simulink model "TailsitterSimModel_ArduPilot_SITL"  (R2018b)
settings: Solver=ode23  StartTime=0  StopTime=1200  FixedStep=0.01  RelTol=1e-4  EnableMultiTasking=on
undefined symbols (not defined in the file): envir
libraries: unit_conversions_lib x3, tailsitter_lib x2, ardupilot_sitl_lib x2, atmosphere_lib x1, flightgear_visualization_lib x1, actuators_lib x1, sensors_lib x1
settings Model: EnablePacing=on  Creator=Yannic  LastModifiedBy=yannic
settings SolverCC: ZeroCrossControl=DisableAll  AlgebraicLoopSolver=LineSearch
settings DataIOCC: LimitDataPoints=on  SaveFormat=StructureWithTime
settings OptimizationCC: BlockReduction=off  DefaultParameterBehavior=Inlined  DefaultUnderspecifiedDataType=single  OptimizeBlockIOStorage=off  BufferReuse=off  GlobalBufferReuse=off  ExpressionFolding=off  LocalBlockOutputs=off  LifeSpan=inf  OptimizeDataStoreBuffers=off  BusAssignmentInplaceUpdate=off
settings DebuggingCC: AlgebraicLoopMsg=none  UnconnectedInputMsg=none  UnconnectedOutputMsg=none  UnconnectedLineMsg=none  AllowSymbolicDim=off  SFUnexpectedBacktrackingDiag=warning  SFNoUnconditionalDefaultTransitionDiag=warning  SFExecutionAtInitializationDiag=none
settings ModelReferenceCC: PropagateSignalLabelsOutOfModel=off
settings SFSimCC: SimUseLocalCustomCode=off
settings RTWCC: RTWUseLocalCustomCode=off
settings CodeAppCC: StateflowObjectComments=on
settings GRTTargetCC: TargetLangStandard=C89/C90 (ANSI)
settings ConfigComp: CovMetricSettings=dw  CovHtmlReporting=on  CovSaveCumulativeToWorkspaceVar=on  CovSaveSingleToWorkspaceVar=on  CovExternalEMLEnable=off

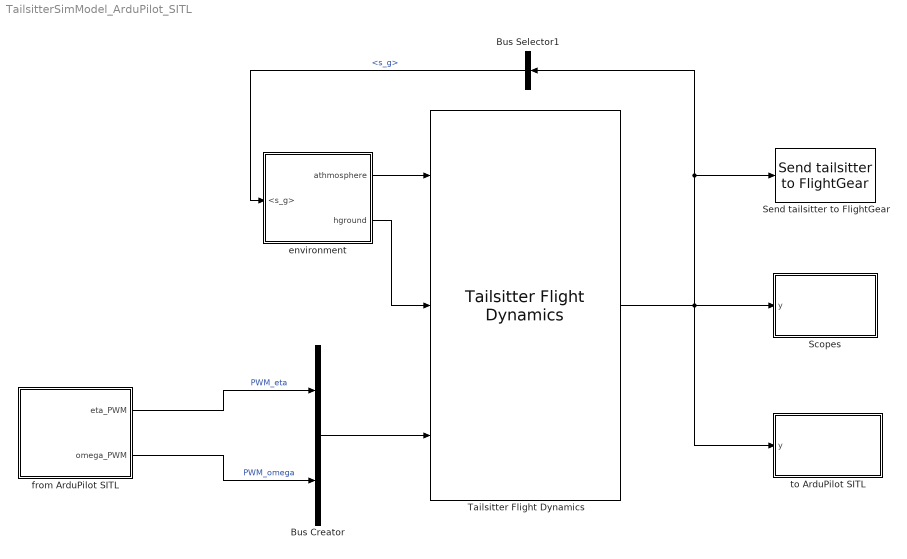
== system TailsitterSimModel_ArduPilot_SITL ==
  Bus Creator : BusCreator  Inputs=2
  Bus Selector1 : BusSelector  OutputSignals=rigid_body.s_g
  Scopes : Subsystem
  Send tailsitter to FlightGear : tailsitter_lib/Send tailsitter to FlightGear  posRef=tailsitter.posRef  IP='127.0.0.1'  Port=5502
      settings: SourceProductName=LADAC
  Tailsitter Flight Dynamics : tailsitter_lib/Tailsitter Flight Dynamics  tailsitter=tailsitter
      settings: SourceProductName=LADAC
  environment : Subsystem
  from ArduPilot SITL : Subsystem
  to ArduPilot SITL : Subsystem
  wires:
  from ArduPilot SITL/2(omega_PWM) -> Bus Creator/2  "PWM_omega"
  from ArduPilot SITL/1(eta_PWM) -> Bus Creator/1  "PWM_eta"
  Bus Creator/1 -> Tailsitter Flight Dynamics/3
  environment/1(athmosphere) -> Tailsitter Flight Dynamics/1
  environment/2(hground) -> Tailsitter Flight Dynamics/2
  Tailsitter Flight Dynamics/1 -> Send tailsitter to FlightGear/1, Bus Selector1/1, Scopes/1(y), to ArduPilot SITL/1(y)
  Bus Selector1/1 -> environment/1(<s_g>)  "<s_g>"

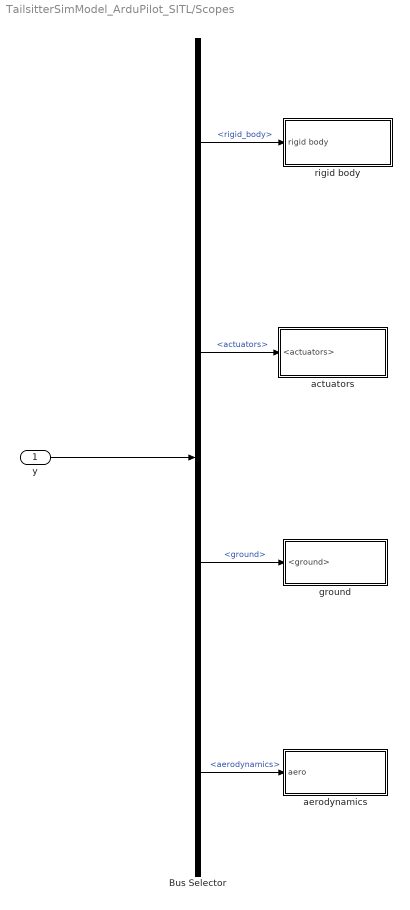
== system TailsitterSimModel_ArduPilot_SITL/Scopes ==
  y : Inport
  Bus Selector : BusSelector  OutputSignals=rigid_body,actuators,ground,aerodynamics
  actuators : Subsystem
  aerodynamics : Subsystem
  ground : Subsystem
  rigid body : Subsystem
  wires:
  Bus Selector/1 -> rigid body/1(rigid body)  "<rigid_body>"
  y/1 -> Bus Selector/1
  Bus Selector/4 -> aerodynamics/1(aero)  "<aerodynamics>"
  Bus Selector/3 -> ground/1(<ground>)  "<ground>"
  Bus Selector/2 -> actuators/1(<actuators>)  "<actuators>"

== system TailsitterSimModel_ArduPilot_SITL/environment ==
  <s_g> : Inport
  Atmosphere1 : Subsystem
  From FlightGear : Subsystem
  athmosphere : Outport
  hground : Outport  Port=2
  wires:
  From FlightGear/1(hground) -> hground/1
  Atmosphere1/1(atmosphere) -> athmosphere/1
  <s_g>/1 -> Atmosphere1/1(s_g)

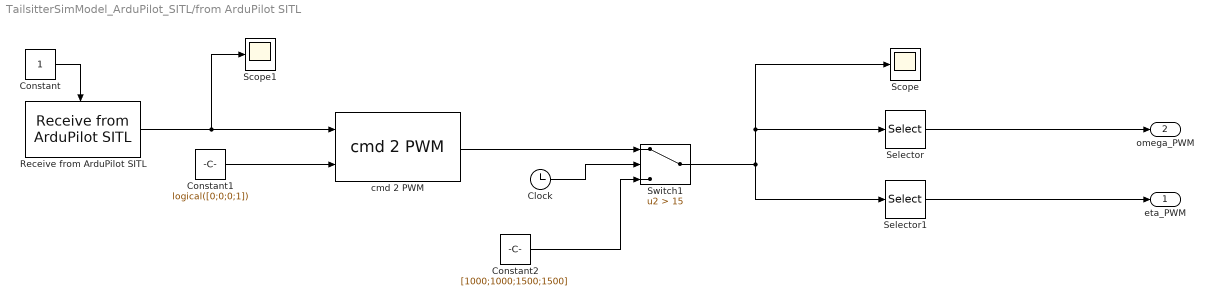
== system TailsitterSimModel_ArduPilot_SITL/from ArduPilot SITL ==
  Clock : Clock
  Constant : Constant  OutDataTypeStr=boolean
  Constant1 : Constant  Value=logical([0;0;0;1])
  Constant2 : Constant  Value=[1000;1000;1500;1500]
  Receive from ArduPilot SITL : ardupilot_sitl_lib/Receive from ArduPilot SITL  idx=[2,1,6,5]  IP='127.0.0.1'  Port=9002  sample_time=SITL.sample_time  blocking_time=1
      settings: SourceProductName=LADAC
  Scope : Scope
  Scope1 : Scope
  Selector : Selector  InputPortWidth=4  IndexOptions=Index vector (dialog)  Indices=[1,2]  OutputSizes=1
  Selector1 : Selector  InputPortWidth=4  IndexOptions=Index vector (dialog)  Indices=[3,4]  OutputSizes=1
  Switch1 : Switch  Criteria=u2 > Threshold  Threshold=15
  cmd 2 PWM : actuators_lib/cmd 2 PWM  SystemSampleTime=-1
      settings: SourceProductName=LADAC
  eta_PWM : Outport
  omega_PWM : Outport  Port=2
  wires:
  Constant2/1 -> Switch1/3
  Constant1/1 -> cmd 2 PWM/2
  Selector/1 -> omega_PWM/1
  cmd 2 PWM/1 -> Switch1/1
  Selector1/1 -> eta_PWM/1
  Receive from ArduPilot SITL/1 -> cmd 2 PWM/1, Scope1/1
  Clock/1 -> Switch1/2
  Switch1/1 -> Selector1/1, Scope/1, Selector/1
  Constant/1 -> Receive from ArduPilot SITL/Enable

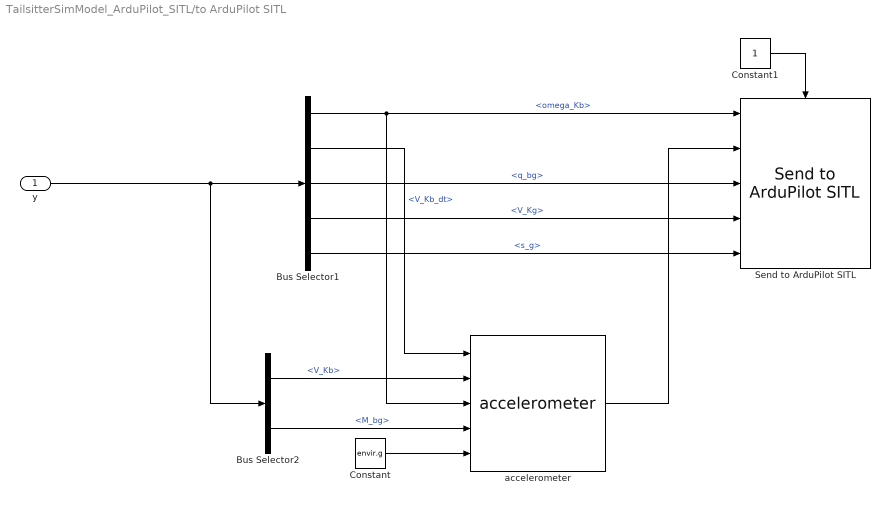
== system TailsitterSimModel_ArduPilot_SITL/to ArduPilot SITL ==
  y : Inport
  Bus Selector1 : BusSelector  OutputSignals=rigid_body.omega_Kb,rigid_body.V_Kb_dt,rigid_body.q_bg,rigid_body.V_Kg,rigid_body.s_g
  Bus Selector2 : BusSelector  OutputSignals=rigid_body.V_Kb,rigid_body.M_bg
  Constant : Constant  Value=envir.g
  Constant1 : Constant  OutDataTypeStr=boolean
  Send to ArduPilot SITL : ardupilot_sitl_lib/Send to ArduPilot SITL  IP='127.0.0.1'  Port=9003  sample_time=SITL.sample_time
      settings: SourceProductName=LADAC
  accelerometer : sensors_lib/accelerometer  SystemSampleTime=-1
      settings: SourceProductName=LADAC
  wires:
  Bus Selector1/5 -> Send to ArduPilot SITL/5  "<s_g>"
  Constant/1 -> accelerometer/5
  y/1 -> Bus Selector1/1, Bus Selector2/1
  Bus Selector2/1 -> accelerometer/2  "<V_Kb>"
  Bus Selector1/2 -> accelerometer/1  "<V_Kb_dt>"
  Bus Selector2/2 -> accelerometer/4  "<M_bg>"
  accelerometer/1 -> Send to ArduPilot SITL/2
  Bus Selector1/3 -> Send to ArduPilot SITL/3  "<q_bg>"
  Bus Selector1/4 -> Send to ArduPilot SITL/4  "<V_Kg>"
  Bus Selector1/1 -> accelerometer/3, Send to ArduPilot SITL/1  "<omega_Kb>"
  Constant1/1 -> Send to ArduPilot SITL/Enable

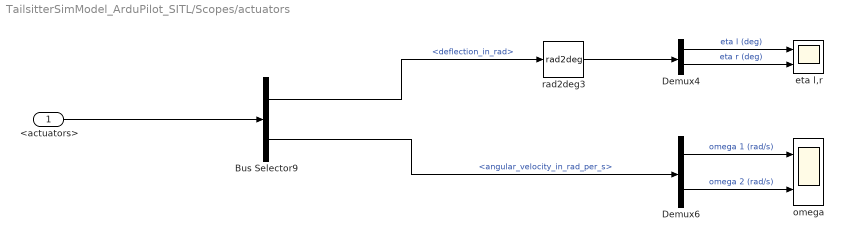
== system TailsitterSimModel_ArduPilot_SITL/Scopes/actuators ==
  <actuators> : Inport
  Bus Selector9 : BusSelector  OutputSignals=eta_i.deflection_in_rad,angular_velocity_in_rad_per_s
  Demux4 : Demux  Outputs=2
  Demux6 : Demux  Outputs=2
  eta l,r : Scope  NumInputPorts=2
  omega : Scope  NumInputPorts=2
  rad2deg3 : unit_conversions_lib/rad2deg
      settings: SourceProductName=LADAC
  wires:
  Bus Selector9/1 -> rad2deg3/1  "<deflection_in_rad>"
  Demux4/1 -> eta l,r/1  "eta l (deg)"
  <actuators>/1 -> Bus Selector9/1
  Demux6/2 -> omega/2  "omega 2 (rad/s)"
  Demux4/2 -> eta l,r/2  "eta r (deg)"
  rad2deg3/1 -> Demux4/1
  Demux6/1 -> omega/1  "omega 1 (rad/s)"
  Bus Selector9/2 -> Demux6/1  "<angular_velocity_in_rad_per_s>"

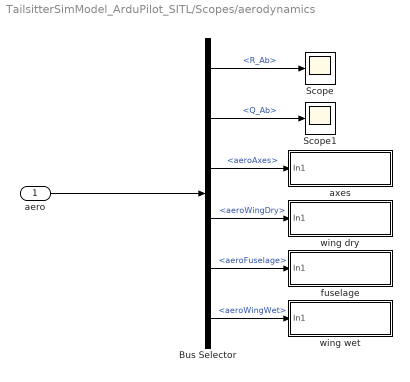
== system TailsitterSimModel_ArduPilot_SITL/Scopes/aerodynamics ==
  aero : Inport
  Bus Selector : BusSelector  OutputSignals=cg aerodynamics.R_Ab,cg aerodynamics.Q_Ab,cg aerodynamics.aeroAxes,local aerodynamic.aeroWingDry,local aerodynamic.aeroFuselage,local aerodynamic.aeroWingWet
  Scope : Scope
  Scope1 : Scope
  axes : Subsystem
  fuselage : Subsystem
  wing dry : Subsystem
  wing wet : Subsystem
  wires:
  aero/1 -> Bus Selector/1
  Bus Selector/1 -> Scope/1  "<R_Ab>"
  Bus Selector/2 -> Scope1/1  "<Q_Ab>"
  Bus Selector/3 -> axes/1(In1)  "<aeroAxes>"
  Bus Selector/4 -> wing dry/1(In1)  "<aeroWingDry>"
  Bus Selector/5 -> fuselage/1(In1)  "<aeroFuselage>"
  Bus Selector/6 -> wing wet/1(In1)  "<aeroWingWet>"

== system TailsitterSimModel_ArduPilot_SITL/Scopes/ground ==
  <ground> : Inport
  Bus Selector1 : BusSelector  Commented=on  OutputSignals=R_Gb,Q_Gb,alt_hitpoints,e_z
  Scope{1..4} (4 alike) : Scope  Commented=on
  wires:
  <ground>/1 -> Bus Selector1/1
  Bus Selector1/2 -> Scope2/1  "<Q_Gb>"
  Bus Selector1/3 -> Scope3/1  "<alt_hitpoints>"
  Bus Selector1/1 -> Scope1/1  "<R_Gb>"
  Bus Selector1/4 -> Scope4/1  "<e_z>"

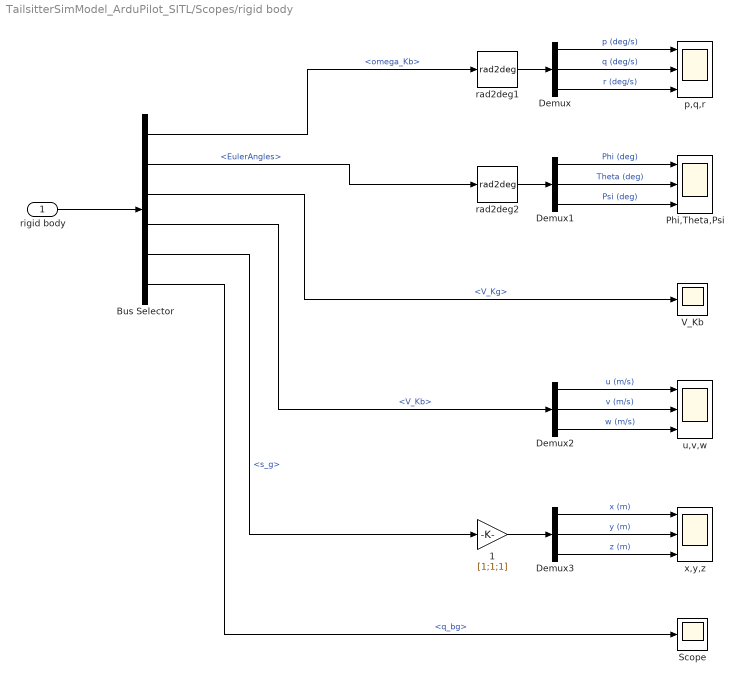
== system TailsitterSimModel_ArduPilot_SITL/Scopes/rigid body ==
  rigid body : Inport
  1 : Gain  Gain=[1;1;1]
  Bus Selector : BusSelector  OutputSignals=omega_Kb,EulerAngles,V_Kg,V_Kb,s_g,q_bg
  Demux{,1..3} (4 alike) : Demux  Outputs=3
  Phi,Theta,Psi : Scope  NumInputPorts=3
  Scope : Scope
  V_Kb : Scope
  p,q,r : Scope  NumInputPorts=3
  rad2deg1 : unit_conversions_lib/rad2deg
      settings: SourceProductName=LADAC
  rad2deg2 : unit_conversions_lib/rad2deg
      settings: SourceProductName=LADAC
  u,v,w : Scope  NumInputPorts=3
  x,y,z : Scope  NumInputPorts=3
  wires:
  rad2deg2/1 -> Demux1/1
  Demux1/3 -> Phi,Theta,Psi/3  "Psi (deg)"
  Demux/3 -> p,q,r/3  "r (deg/s)"
  Demux2/2 -> u,v,w/2  "v (m/s)"
  Demux3/1 -> x,y,z/1  "x (m)"
  Demux2/3 -> u,v,w/3  "w (m/s)"
  rad2deg1/1 -> Demux/1
  Demux/2 -> p,q,r/2  "q (deg/s)"
  Demux2/1 -> u,v,w/1  "u (m/s)"
  Demux/1 -> p,q,r/1  "p (deg/s)"
  1/1 -> Demux3/1
  Bus Selector/3 -> V_Kb/1  "<V_Kg>"
  Demux1/2 -> Phi,Theta,Psi/2  "Theta (deg)"
  Demux3/2 -> x,y,z/2  "y (m)"
  Demux3/3 -> x,y,z/3  "z (m)"
  Demux1/1 -> Phi,Theta,Psi/1  "Phi (deg)"
  rigid body/1 -> Bus Selector/1
  Bus Selector/1 -> rad2deg1/1  "<omega_Kb>"
  Bus Selector/2 -> rad2deg2/1  "<EulerAngles>"
  Bus Selector/4 -> Demux2/1  "<V_Kb>"
  Bus Selector/5 -> 1/1  "<s_g>"
  Bus Selector/6 -> Scope/1  "<q_bg>"

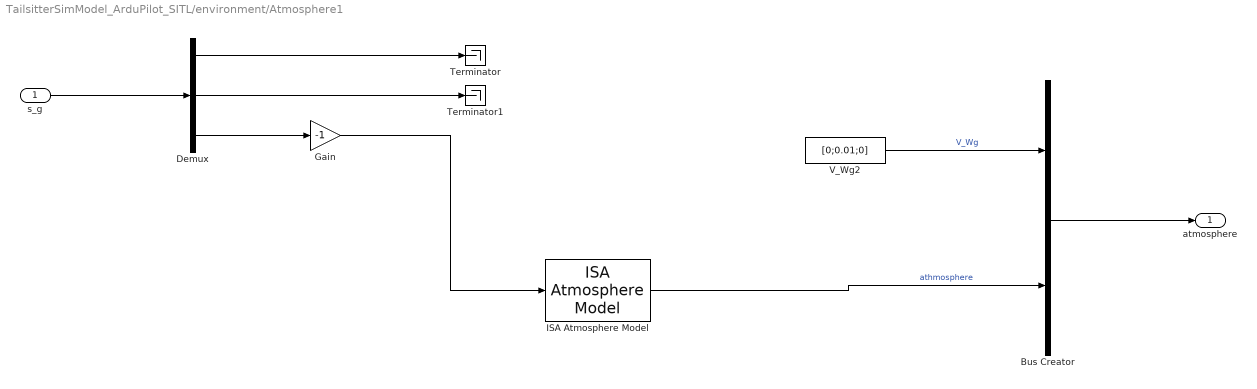
== system TailsitterSimModel_ArduPilot_SITL/environment/Atmosphere1 ==
  s_g : Inport
  Bus Creator : BusCreator  Inputs=2
  Demux : Demux  Outputs=3
  Gain : Gain  Gain=-1
  ISA Atmosphere Model : atmosphere_lib/ISA Atmosphere Model  SystemSampleTime=-1
      settings: SourceProductName=LADAC
  Terminator : Terminator
  Terminator1 : Terminator
  V_Wg2 : Constant  Value=[0;0.01;0]
  atmosphere : Outport
  wires:
  ISA Atmosphere Model/1 -> Bus Creator/2  "athmosphere"
  Demux/1 -> Terminator/1
  Demux/2 -> Terminator1/1
  s_g/1 -> Demux/1
  Demux/3 -> Gain/1
  Gain/1 -> ISA Atmosphere Model/1
  Bus Creator/1 -> atmosphere/1
  V_Wg2/1 -> Bus Creator/1  "V_Wg"

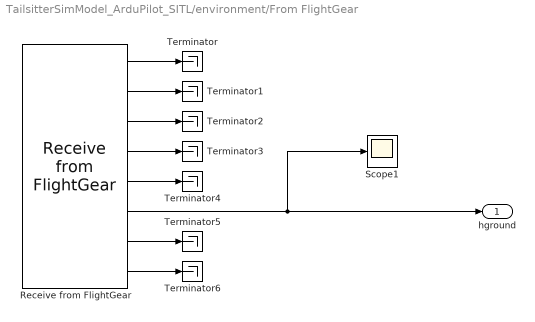
== system TailsitterSimModel_ArduPilot_SITL/environment/From FlightGear ==
  Receive from FlightGear : flightgear_visualization_lib/Receive from FlightGear  ip_address='127.0.0.1'  ip_port=5503  sample_time=1/30  blocking_time=0  is_aerocntrl=off  is_engine=off  is_fuel=off  is_land=off  is_avionics=off  is_envir=on
      settings: SourceProductName=LADAC
  Scope1 : Scope
  Terminator{,1..6} (7 alike) : Terminator
  hground : Outport
  wires:
  Receive from FlightGear/5 -> Terminator4/1
  Receive from FlightGear/4 -> Terminator3/1
  Receive from FlightGear/2 -> Terminator1/1
  Receive from FlightGear/1 -> Terminator/1
  Receive from FlightGear/8 -> Terminator6/1
  Receive from FlightGear/6 -> Scope1/1, hground/1
  Receive from FlightGear/3 -> Terminator2/1
  Receive from FlightGear/7 -> Terminator5/1

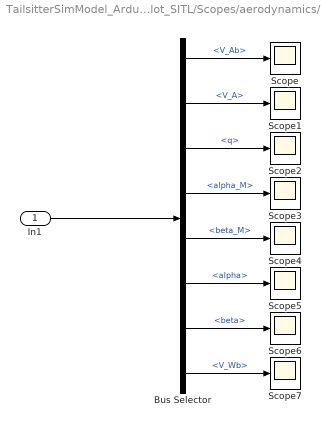
== system TailsitterSimModel_ArduPilot_SITL/Scopes/aerodynamics/axes ==
  In1 : Inport
  Bus Selector : BusSelector  OutputSignals=V_Ab,V_A,q,alpha_M,beta_M,alpha,beta,V_Wb
  Scope{,1..7} (8 alike) : Scope
  wires:
  In1/1 -> Bus Selector/1
  Bus Selector/1 -> Scope/1  "<V_Ab>"
  Bus Selector/2 -> Scope1/1  "<V_A>"
  Bus Selector/3 -> Scope2/1  "<q>"
  Bus Selector/4 -> Scope3/1  "<alpha_M>"
  Bus Selector/5 -> Scope4/1  "<beta_M>"
  Bus Selector/6 -> Scope5/1  "<alpha>"
  Bus Selector/7 -> Scope6/1  "<beta>"
  Bus Selector/8 -> Scope7/1  "<V_Wb>"

== system TailsitterSimModel_ArduPilot_SITL/Scopes/aerodynamics/fuselage ==
  In1 : Inport
  Bus Selector : BusSelector  OutputSignals=aeroAxes,dynamics
  wing weet : Subsystem
  wing weet1 : Subsystem
  wires:
  In1/1 -> Bus Selector/1
  Bus Selector/1 -> wing weet/1(In1)  "<aeroAxes>"
  Bus Selector/2 -> wing weet1/1(In1)  "<dynamics>"

== system TailsitterSimModel_ArduPilot_SITL/Scopes/aerodynamics/wing dry ==
  In1 : Inport
  Bus Selector : BusSelector  OutputSignals=aeroAxes,dynamicsBody
  axes : Subsystem
  dynamics : Subsystem
  wires:
  In1/1 -> Bus Selector/1
  Bus Selector/2 -> dynamics/1(In1)  "<dynamicsBody>"
  Bus Selector/1 -> axes/1(In1)  "<aeroAxes>"

== system TailsitterSimModel_ArduPilot_SITL/Scopes/aerodynamics/wing wet ==
  In1 : Inport
  Bus Selector : BusSelector  OutputSignals=dynamicsBody,aeroAxes
  axes : Subsystem
  dynamics : Subsystem
  wires:
  In1/1 -> Bus Selector/1
  Bus Selector/1 -> dynamics/1(In1)  "<dynamicsBody>"
  Bus Selector/2 -> axes/1(In1)  "<aeroAxes>"

== system TailsitterSimModel_ArduPilot_SITL/Scopes/aerodynamics/fuselage/wing weet ==
  In1 : Inport
  Bus Selector : BusSelector  OutputSignals=V_A_Pfuse,q_Pfuse,alpha_M_Pfuse,beta_M_Pfuse
  Scope{,1..3} (4 alike) : Scope
  wires:
  In1/1 -> Bus Selector/1
  Bus Selector/1 -> Scope/1  "<V_A_Pfuse>"
  Bus Selector/2 -> Scope1/1  "<q_Pfuse>"
  Bus Selector/3 -> Scope2/1  "<alpha_M_Pfuse>"
  Bus Selector/4 -> Scope3/1  "<beta_M_Pfuse>"

== system TailsitterSimModel_ArduPilot_SITL/Scopes/aerodynamics/fuselage/wing weet1 ==
  In1 : Inport
  wires:
  In1/1 -> ?

== system TailsitterSimModel_ArduPilot_SITL/Scopes/aerodynamics/wing dry/axes ==
  In1 : Inport
  Bus Selector : BusSelector  OutputSignals=V_A_P,q_P,alpha_M_P,beta_M_P
  Scope{,1..3} (4 alike) : Scope
  wires:
  In1/1 -> Bus Selector/1
  Bus Selector/1 -> Scope/1  "<V_A_P>"
  Bus Selector/2 -> Scope1/1  "<q_P>"
  Bus Selector/3 -> Scope2/1  "<alpha_M_P>"
  Bus Selector/4 -> Scope3/1  "<beta_M_P>"

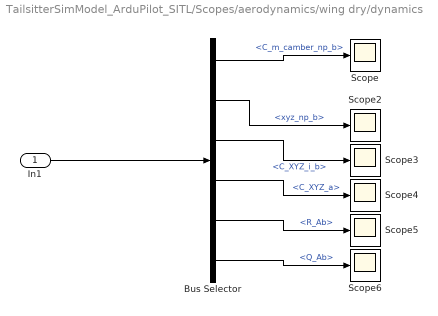
== system TailsitterSimModel_ArduPilot_SITL/Scopes/aerodynamics/wing dry/dynamics ==
  In1 : Inport
  Bus Selector : BusSelector  OutputSignals=C_m_camber_np_b,xyz_np_b,C_XYZ_i_b,C_XYZ_a,R_Ab,Q_Ab
  Scope{,2..6} (6 alike) : Scope
  wires:
  In1/1 -> Bus Selector/1
  Bus Selector/1 -> Scope/1  "<C_m_camber_np_b>"
  Bus Selector/2 -> Scope2/1  "<xyz_np_b>"
  Bus Selector/3 -> Scope3/1  "<C_XYZ_i_b>"
  Bus Selector/4 -> Scope4/1  "<C_XYZ_a>"
  Bus Selector/5 -> Scope5/1  "<R_Ab>"
  Bus Selector/6 -> Scope6/1  "<Q_Ab>"

== system TailsitterSimModel_ArduPilot_SITL/Scopes/aerodynamics/wing wet/axes ==
  In1 : Inport
  Bus Selector : BusSelector  OutputSignals=V_A_P,q_P,alpha_M_P,beta_M_P
  Scope{,1..3} (4 alike) : Scope
  wires:
  In1/1 -> Bus Selector/1
  Bus Selector/1 -> Scope/1  "<V_A_P>"
  Bus Selector/2 -> Scope1/1  "<q_P>"
  Bus Selector/3 -> Scope2/1  "<alpha_M_P>"
  Bus Selector/4 -> Scope3/1  "<beta_M_P>"

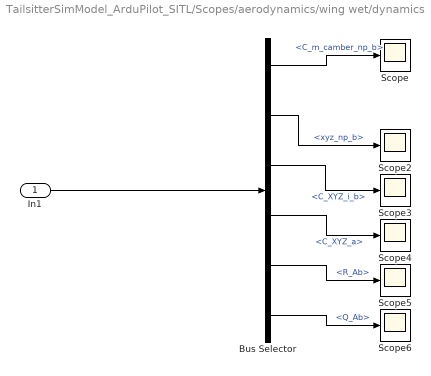
== system TailsitterSimModel_ArduPilot_SITL/Scopes/aerodynamics/wing wet/dynamics ==
  In1 : Inport
  Bus Selector : BusSelector  OutputSignals=C_m_camber_np_b,xyz_np_b,C_XYZ_i_b,C_XYZ_a,R_Ab,Q_Ab
  Scope{,2..6} (6 alike) : Scope
  wires:
  In1/1 -> Bus Selector/1
  Bus Selector/1 -> Scope/1  "<C_m_camber_np_b>"
  Bus Selector/2 -> Scope2/1  "<xyz_np_b>"
  Bus Selector/3 -> Scope3/1  "<C_XYZ_i_b>"
  Bus Selector/4 -> Scope4/1  "<C_XYZ_a>"
  Bus Selector/5 -> Scope5/1  "<R_Ab>"
  Bus Selector/6 -> Scope6/1  "<Q_Ab>"
